simulink model "pipelined_adc_stage_test"  (R2019a)
settings: Solver=FixedStepDiscrete  StartTime=0.0  StopTime=300.0  FixedStep=1  RelTol=1e-3
libraries: pipelined_adc_library x1, simulink x1
settings Model: Creator=johan  LastModifiedBy=johan

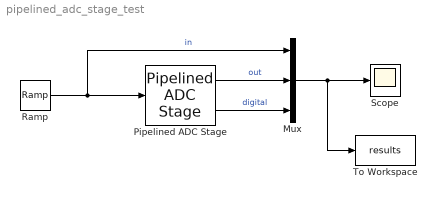
== system pipelined_adc_stage_test ==
  Mux : Mux  Inputs=3
  Pipelined ADC Stage : pipelined_adc_library/Pipelined ADC Stage  comp_offsets=[0, 0, 0, 0, 0, 0]  sigma_noise=0
  Ramp : simulink/Sources/Ramp  slope=0.01  start=0  InitialOutput=-1.5
  Scope : Scope
  To Workspace : ToWorkspace  VariableName=results  SaveFormat=Structure  SampleTime=-1
  wires:
  Mux/1 -> To Workspace/1, Scope/1
  Pipelined ADC Stage/1 -> Mux/2  "out"
  Ramp/1 -> Pipelined ADC Stage/1, Mux/1  "in"
  Pipelined ADC Stage/2 -> Mux/3  "digital"
